simulink model "UAVSimulation"  (R2021b)
settings: Solver=VariableStepAuto  StartTime=0  StopTime=60  RelTol=1e-3
values from neighbouring files (symbols this model uses):
  m = 120000    [UAV_model.m]
  u1max = 25*pi/180    (= 0.436332312999)    [UAV_model.m]    (also in init.m; trim_values_straight_level.mat)
  u1min = -25*pi/180    (= -0.436332312999)    [UAV_model.m]    (also in init.m; trim_values_straight_level.mat)
  u2max = 10*pi/180    (= 0.174532925199)    [UAV_model.m]    (also in init.m; trim_values_straight_level.mat)
  u2min = -25*pi/180    (= -0.436332312999)    [UAV_model.m]    (also in init.m; trim_values_straight_level.mat)
  u4max = 10*pi/180    (= 0.174532925199)    [UAV_model.m]    (also in init.m; trim_values_straight_level.mat)
  u4min = 0.5*pi/180    (= 0.00872664625997)    [UAV_model.m]    (also in init.m; trim_values_straight_level.mat)
  u5max = 10*pi/180    (= 0.174532925199)    [UAV_model.m]    (also in init.m; trim_values_straight_level.mat)
  u5min = 0.5*pi/180    (= 0.00872664625997)    [UAV_model.m]    (also in init.m; trim_values_straight_level.mat)
  UStar = ZStar(10:14)    [UAV_trim.m]    (also in ValidateTrimPoint.m = temp.UStar; init.m = temp.UStar; trim_values_straight_level.mat = [0.000230087416011 -0.178007222496 0.000542025698534 0.08223)
  XStar = ZStar(1:9)    [UAV_trim.m]    (also in ValidateTrimPoint.m = temp.XStar; init.m = temp.XStar; trim_values_straight_level.mat = [84.9904926066 3.96412927226e-06 1.27128425211 2.6281652208e)
undefined symbols (not defined in the file or in its folder): Earth, ft, Payload, Receive, s, Send, UAV_model, WGS84
libraries: aerolibconvert2 x4, uavmavlinklib x4, simulink_extras x3, dspnetwork x3, aerolibfltsims x2, dspsigattribs x2, aerolibtransform2 x2, sensorgpslib x1, uavalgslib x1
settings Model: Creator=mikol  LastModifiedBy=mikol
settings SolverCC: AlgebraicLoopSolver=TrustRegion
settings DataIOCC: SaveFormat=StructureWithTime
settings OptimizationCC: BlockReduction=off  BufferReuse=off
settings DebuggingCC: AlgebraicLoopMsg=none  UnconnectedInputMsg=none  UnconnectedOutputMsg=none  UnconnectedLineMsg=none  SFMachineParentedDataDiag=warning
settings ExplorerConfigSet: SimMechanicsOpenEditorOnUpdate=off

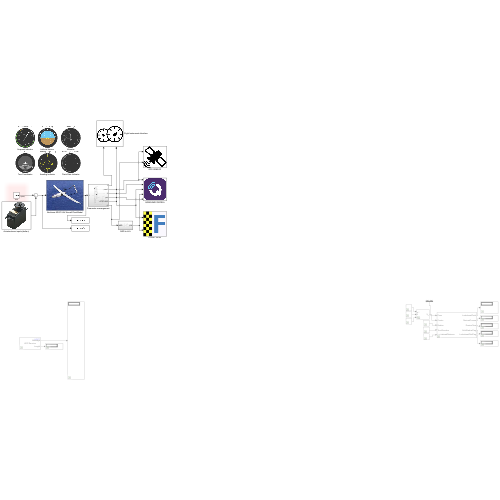
[thumbnail: Simulink's stored preview of the top-level diagram]
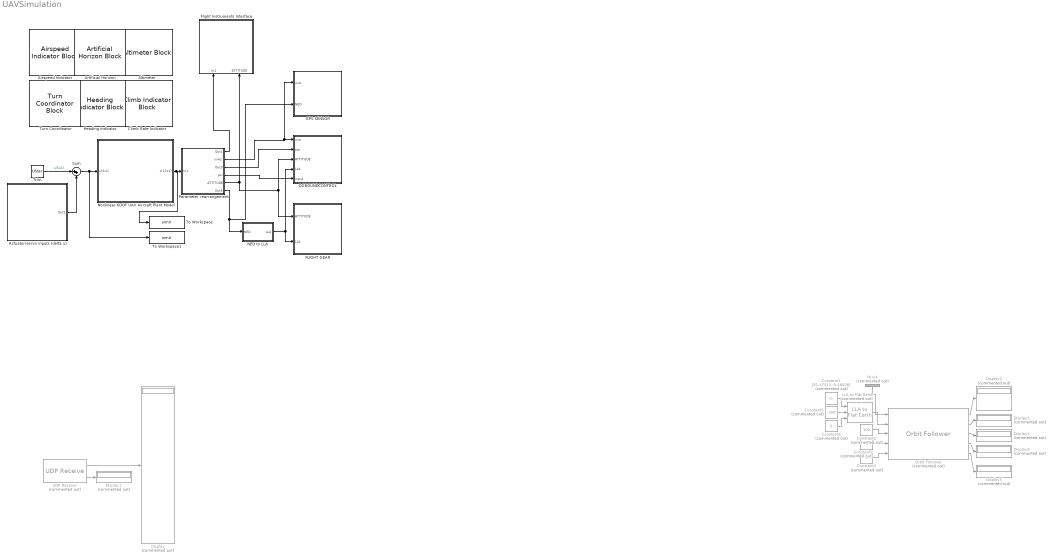
== system UAVSimulation ==
  Actuator/servo inputs (delta u) : Subsystem
      mask Display: image('FUTM0075_A0_R28XQZ28.jpg'); % Use "Edit Image" on toolstrip to change.
  Airspeed Indicator : AirspeedIndicatorBlock
  Altimeter : AltimeterBlock
  Artificial Horizon : ArtificialHorizonBlock
  Climb Rate Indicator : ClimbIndicatorBlock
  Constant1 : Constant  Commented=on  Value=[51.47413 -0.46008]
  Constant2 : Constant  Commented=on  Value=100
  Constant3 : Constant  Commented=on
  Constant4 : Constant  Commented=on  Value=5
  Constant5 : Constant  Commented=on  Value=-300
  Constant6 : Constant  Commented=on  Value=0
  Display{,1..6} (7 alike) : Display  Commented=on
  FLIGHT GEAR : Subsystem
      mask Display: image('icon.png'); % Use "Edit Image" on toolstrip to change.
  Flight Instruments Interface : Subsystem
      mask Display: image('167346-200.png'); % Use "Edit Image" on toolstrip to change.
  GPS SENSOR : Subsystem
      mask Display: image('gps.png'); % Use "Edit Image" on toolstrip to change.
  Heading Indicator : HeadingIndicatorBlock
  LLA to Flat Earth : aerolibtransform2/LLA to Flat Earth  Commented=on  units=Metric (MKS)  ptype=Earth (WGS84)  F=1/298.257223563  R=6378137  refPosPort=off  LL0=[51.47413 -0.46008]  psi=0
      settings: SourceProductBaseCode=AE
  Mux4 : Mux  Commented=on  Inputs=2
  NED to LLA : Subsystem
  Nonlinear 6DOF UAV Aircraft Plant Model : Subsystem
      mask Display: image('aerosonde-uav-bg.jpg'); % Use "Edit Image" on toolstrip to change.
  Orbit Follower : uavalgslib/Orbit Follower  Commented=on  UAVType=fixed-wing  MinOrbitRadius=1  MinLookaheadDistance=0.1  ExternalReset=none  ShowCrossTrackErrorOutput=off  ShowNumTurnsOutput=off  SimulateUsing=Interpreted execution
      settings: SourceProductBaseCode=UV
  Parameter rearrangement : Subsystem
  QGROUNDCONTROL : Subsystem
      mask Display: image('QGroundControl_App_Icon.png'); % Use "Edit Image" on toolstrip to change.
  Sum : Sum  Inputs=|++
  To Workspace : ToWorkspace  VariableName=simX  SaveFormat=Timeseries  SampleTime=-1
  To Workspace1 : ToWorkspace  VariableName=simU  SaveFormat=Timeseries  SampleTime=-1
  Trim : Constant  Value=UStar
  Turn Coordinator : TurnCoordinatorBlock
  UDP Receive : dspnetwork/UDP Receive  Commented=on  localURL='0.0.0.0'  localPort=14500  remoteURL='0.0.0.0'  remotePort=-1  recvBufferSize=8192  dims=263  signalDatatype=uint8  isComplex=off  isVarSize=off  showBlockingTime=on  blockingTime=0  sampletime=0.01  blockPlatform=HOST
  wires:
  Nonlinear 6DOF UAV Aircraft Plant Model/1(x(12x1)) -> To Workspace/1, Parameter rearrangement/1(In1)
  Trim/1 -> Sum/1  "u(5x1)"
  Actuator/servo inputs (delta u)/1(Out1) -> Sum/2
  Sum/1 -> To Workspace1/1, Nonlinear 6DOF UAV Aircraft Plant Model/1(u(5x1))
  UDP Receive/1 -> Display/1
  UDP Receive/2 -> Display1/1
  Mux4/1 -> Orbit Follower/1
  Constant4/1 -> Orbit Follower/5
  Orbit Follower/3 -> Display4/1
  Orbit Follower/1 -> Display2/1
  Orbit Follower/4 -> Display6/1
  Constant3/1 -> Orbit Follower/4
  Orbit Follower/2 -> Display3/1
  Constant5/1 -> LLA to Flat Earth/2
  Constant1/1 -> LLA to Flat Earth/1
  LLA to Flat Earth/1 -> Orbit Follower/2
  Constant2/1 -> Orbit Follower/3
  Orbit Follower/5 -> Display5/1
  Constant6/1 -> LLA to Flat Earth/3
  NED to LLA/1(LLA) -> FLIGHT GEAR/2(LLA), QGROUNDCONTROL/4(LLA)
  Parameter rearrangement/5(ATTITUDE) -> Flight Instruments Interface/2(ATTITUDE), FLIGHT GEAR/1(ATTITUDE), QGROUNDCONTROL/3(ATTITUDE)
  Parameter rearrangement/2(uvw1) -> GPS SENSOR/1(uvw), QGROUNDCONTROL/1(uvw)
  Parameter rearrangement/6(Out6) -> GPS SENSOR/2(NED), NED to LLA/1(NED)
  Parameter rearrangement/1(Out1) -> Flight Instruments Interface/1(In1)
  Parameter rearrangement/3(Out3) -> QGROUNDCONTROL/2(pqr)
  Parameter rearrangement/4(psi) -> QGROUNDCONTROL/5(Input)

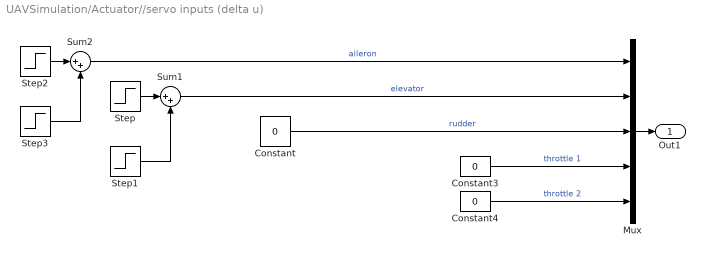
== system UAVSimulation/Actuator//servo inputs (delta u) ==
  Constant : Constant  Value=0
  Constant3 : Constant  Value=0
  Constant4 : Constant  Value=0
  Mux : Mux  Inputs=5
  Step : Step  Time=10  After=-5*pi/180  SampleTime=0
  Step1 : Step  Time=10+5  After=5*pi/180  SampleTime=0
  Step2 : Step  Time=15  After=-5*pi/180  SampleTime=0
  Step3 : Step  Time=15+20  After=5*pi/180  SampleTime=0
  Sum1 : Sum  Inputs=|++
  Sum2 : Sum  Inputs=|++
  Out1 : Outport
  wires:
  Step/1 -> Sum1/1
  Constant/1 -> Mux/3  "rudder"
  Constant4/1 -> Mux/5  "throttle 2"
  Step1/1 -> Sum1/2
  Constant3/1 -> Mux/4  "throttle 1"
  Mux/1 -> Out1/1
  Sum2/1 -> Mux/1  "aileron"
  Sum1/1 -> Mux/2  "elevator"
  Step2/1 -> Sum2/1
  Step3/1 -> Sum2/2

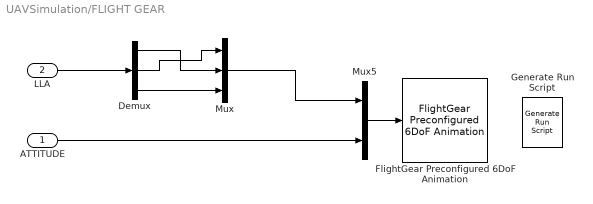
== system UAVSimulation/FLIGHT GEAR ==
  ATTITUDE : Inport
  LLA : Inport  Port=2
  Demux : Demux  Outputs=3
  FlightGear Preconfigured 6DoF Animation : aerolibfltsims/FlightGear Preconfigured 6DoF Animation  xFlightGearVersion=v2019.1  DestinationIpAddress=127.0.0.1  DestinationPort=5502  SampleTime=1/30  packetVersion=24
  Generate Run Script : aerolibfltsims/Generate Run Script  Architecture=Win64  dataFlow=Send-Receive  GeometryModelName=c172p  AirportId=KSFO  RunwayId=10L  InitialAltitude=7224  InitialHeading=113  OffsetDistance=4.72  OffsetAzimuth=0  InstallScenery=on  DisableShaders=on  OriginAddress=127.0.0.1  DestinationPort=5502  OriginPort=5505  LocalAddress=127.0.0.1  OutputFileName=runfg.bat  FlightGearBaseDirectory=D:\Program Files\FlightGear 2020.3
  Mux : Mux  Inputs=3
  Mux5 : Mux  Inputs=2
  wires:
  Mux5/1 -> FlightGear Preconfigured 6DoF Animation/1
  ATTITUDE/1 -> Mux5/2
  Mux/1 -> Mux5/1
  LLA/1 -> Demux/1
  Demux/1 -> Mux/2
  Demux/2 -> Mux/1
  Demux/3 -> Mux/3

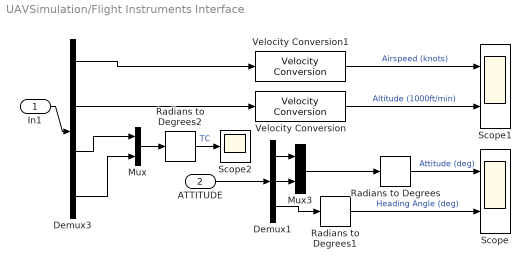
== system UAVSimulation/Flight Instruments Interface ==
  In1 : Inport
  ATTITUDE : Inport  Port=2
  Demux1 : Demux  Outputs=3
  Demux3 : Demux
  Mux : Mux  Inputs=2
  Mux3 : Mux  Inputs=2
  Radians to Degrees : simulink_extras/Transformations/Radians to Degrees
  Radians to Degrees1 : simulink_extras/Transformations/Radians to Degrees
  Radians to Degrees2 : simulink_extras/Transformations/Radians to Degrees
  Scope : Scope  NumInputPorts=2
  Scope1 : Scope  NumInputPorts=2
  Scope2 : Scope
  Velocity Conversion : aerolibconvert2/Velocity Conversion  IU=m/s  OU=ft/min
  Velocity Conversion1 : aerolibconvert2/Velocity Conversion  IU=m/s  OU=kts
  wires:
  Velocity Conversion1/1 -> Scope1/1  "Airspeed (knots)"
  Demux1/2 -> Mux3/2
  In1/1 -> Demux3/1
  Demux1/3 -> Radians to Degrees1/1
  Demux3/2 -> Velocity Conversion/1
  Mux3/1 -> Radians to Degrees/1
  Radians to Degrees/1 -> Scope/1  "Attitude (deg)"
  Radians to Degrees1/1 -> Scope/2  "Heading Angle (deg)"
  Velocity Conversion/1 -> Scope1/2  "Altitude (1000ft/min)"
  Demux1/1 -> Mux3/1
  Radians to Degrees2/1 -> Scope2/1  "TC"
  Mux/1 -> Radians to Degrees2/1
  Demux3/3 -> Mux/1
  Demux3/4 -> Mux/2
  Demux3/1 -> Velocity Conversion1/1
  ATTITUDE/1 -> Demux1/1

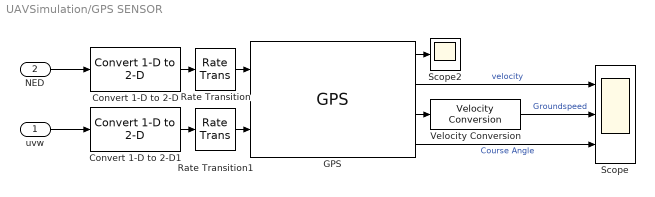
== system UAVSimulation/GPS SENSOR ==
  uvw : Inport
  NED : Inport  Port=2
  Convert 1-D to 2-D : dspsigattribs/Convert 1-D to 2-D  M=1  N=3  frameBasedOut=off
      settings: SourceProductBaseCode=DS
  Convert 1-D to 2-D1 : dspsigattribs/Convert 1-D to 2-D  M=1  N=3  frameBasedOut=off
      settings: SourceProductBaseCode=DS
  GPS : sensorgpslib/GPS  DispRefFrame=NED  PositionInputFormat=Geodetic  ReferenceLocation=[ 0, 0, 0 ]  HorizontalPositionAccuracy=1.6  VerticalPositionAccuracy=3  VelocityAccuracy=0.1  DecayFactor=0.999  SeedDouble=67  SimulateUsing=Interpreted execution
      settings: SourceProductBaseCode=TF,NV,UV
  Rate Transition : RateTransition  OutPortSampleTime=0.2
  Rate Transition1 : RateTransition  OutPortSampleTime=0.2
  Scope : Scope  NumInputPorts=3
  Scope2 : Scope
  Velocity Conversion : aerolibconvert2/Velocity Conversion  IU=m/s  OU=kts
  wires:
  GPS/3 -> Velocity Conversion/1
  Convert 1-D to 2-D/1 -> Rate Transition/1
  Rate Transition1/1 -> GPS/2
  GPS/1 -> Scope2/1
  Rate Transition/1 -> GPS/1
  GPS/4 -> Scope/3  "Course Angle"
  Convert 1-D to 2-D1/1 -> Rate Transition1/1
  GPS/2 -> Scope/1  "velocity"
  Velocity Conversion/1 -> Scope/2  "Groundspeed"
  uvw/1 -> Convert 1-D to 2-D1/1
  NED/1 -> Convert 1-D to 2-D/1

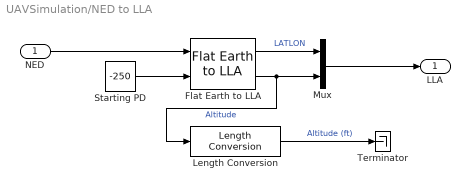
== system UAVSimulation/NED to LLA ==
  NED : Inport
  Flat Earth to LLA : aerolibtransform2/Flat Earth to LLA  units=Metric (MKS)  ptype=Earth (WGS84)  F=1/298.257223563  R=6378137  refPosPort=off  LL0=[51.47413 -0.46008]  psi=0
  Length Conversion : aerolibconvert2/Length Conversion  IU=m  OU=ft
  Mux : Mux  Inputs=2
  Starting PD : Constant  Value=-250
  Terminator : Terminator
  LLA : Outport
  wires:
  Starting PD/1 -> Flat Earth to LLA/2
  NED/1 -> Flat Earth to LLA/1
  Flat Earth to LLA/1 -> Mux/1  "LATLON"
  Flat Earth to LLA/2 -> Length Conversion/1, Mux/2  "Altitude"
  Mux/1 -> LLA/1
  Length Conversion/1 -> Terminator/1  "Altitude (ft)"

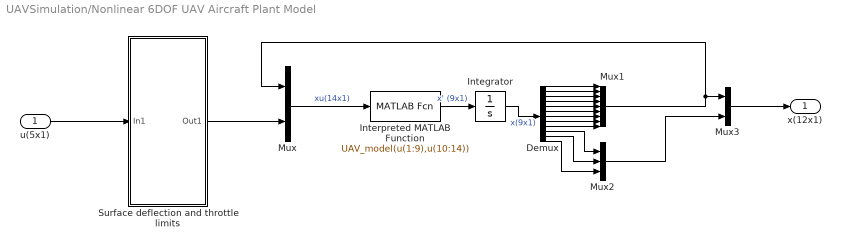
== system UAVSimulation/Nonlinear 6DOF UAV Aircraft Plant Model ==
  u(5x1) : Inport
  Demux : Demux  Outputs=12
  Integrator : Integrator  InitialCondition=XStar
  Interpreted MATLAB Function : MATLABFcn  MATLABFcn=UAV_model(u(1:9),u(10:14))
  Mux : Mux  Inputs=2
  Mux1 : Mux  Inputs=9
  Mux2 : Mux  Inputs=3
  Mux3 : Mux  Inputs=2
  Surface deflection and throttle limits : Subsystem
  x(12x1) : Outport
  wires:
  Mux/1 -> Interpreted MATLAB Function/1  "xu(14x1)"
  Interpreted MATLAB Function/1 -> Integrator/1  "x' (9x1)"
  u(5x1)/1 -> Surface deflection and throttle limits/1(In1)
  Surface deflection and throttle limits/1(Out1) -> Mux/2
  Demux/1 -> Mux1/1
  Demux/2 -> Mux1/2
  Demux/3 -> Mux1/3
  Demux/4 -> Mux1/4
  Demux/5 -> Mux1/5
  Demux/6 -> Mux1/6
  Demux/7 -> Mux1/7
  Demux/8 -> Mux1/8
  Demux/9 -> Mux1/9
  Demux/10 -> Mux2/1
  Demux/11 -> Mux2/2
  Demux/12 -> Mux2/3
  Mux2/1 -> Mux3/2
  Mux3/1 -> x(12x1)/1
  Integrator/1 -> Demux/1  "x(9x1)"
  Mux1/1 -> Mux/1, Mux3/1

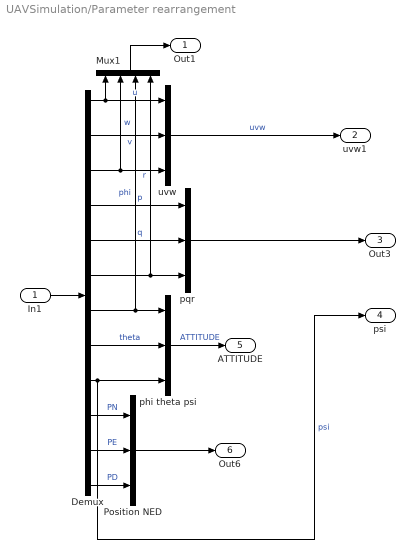
== system UAVSimulation/Parameter rearrangement ==
  In1 : Inport
  Demux : Demux  Outputs=12
  Mux1 : Mux
  Position NED : Mux  Inputs=3
  phi theta psi : Mux  Inputs=3
  pqr : Mux  Inputs=3
  uvw : Mux  Inputs=3
  Out1 : Outport
  uvw1 : Outport  Port=2
  Out3 : Outport  Port=3
  psi : Outport  Port=4
  ATTITUDE : Outport  Port=5
  Out6 : Outport  Port=6
  wires:
  Demux/9 -> phi theta psi/3, psi/1  "psi"
  Demux/5 -> pqr/2  "q"
  Demux/3 -> Mux1/2, uvw/3  "w"
  Demux/10 -> Position NED/1  "PN"
  Demux/1 -> uvw/1, Mux1/1  "u"
  Demux/7 -> phi theta psi/1, Mux1/3  "phi"
  Demux/11 -> Position NED/2  "PE"
  Demux/8 -> phi theta psi/2  "theta"
  Demux/2 -> uvw/2  "v"
  uvw/1 -> uvw1/1  "uvw"
  Demux/12 -> Position NED/3  "PD"
  Demux/4 -> pqr/1  "p"
  Demux/6 -> pqr/3, Mux1/4  "r"
  phi theta psi/1 -> ATTITUDE/1  "ATTITUDE"
  In1/1 -> Demux/1
  pqr/1 -> Out3/1
  Position NED/1 -> Out6/1
  Mux1/1 -> Out1/1

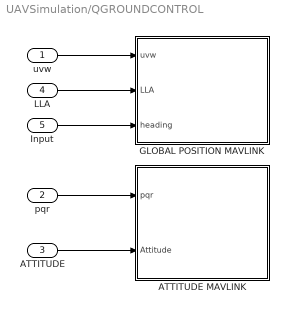
== system UAVSimulation/QGROUNDCONTROL ==
  uvw : Inport
  pqr : Inport  Port=2
  ATTITUDE : Inport  Port=3
  LLA : Inport  Port=4
  Input : Inport  Port=5
  ATTITUDE MAVLINK : Subsystem
  GLOBAL POSITION MAVLINK : Subsystem
  wires:
  uvw/1 -> GLOBAL POSITION MAVLINK/1(uvw)
  pqr/1 -> ATTITUDE MAVLINK/1(pqr)
  ATTITUDE/1 -> ATTITUDE MAVLINK/2(Attitude)
  LLA/1 -> GLOBAL POSITION MAVLINK/2(LLA)
  Input/1 -> GLOBAL POSITION MAVLINK/3(heading)

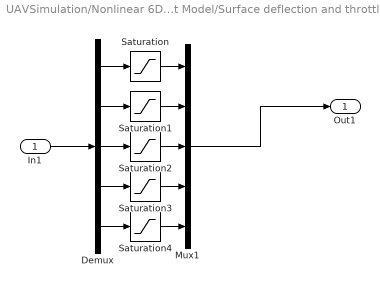
== system UAVSimulation/Nonlinear 6DOF UAV Aircraft Plant Model/Surface deflection and throttle limits ==
  In1 : Inport
  Demux : Demux  Outputs=5
  Mux1 : Mux  Inputs=5
  Saturation : Saturate  UpperLimit=u1max  LowerLimit=u1min
  Saturation1 : Saturate  UpperLimit=u2max  LowerLimit=u2min
  Saturation2 : Saturate  UpperLimit=u1max  LowerLimit=u1min
  Saturation3 : Saturate  UpperLimit=u4max  LowerLimit=u4min
  Saturation4 : Saturate  UpperLimit=u5max  LowerLimit=u5min
  Out1 : Outport
  wires:
  Demux/2 -> Saturation1/1
  Demux/3 -> Saturation2/1
  Saturation3/1 -> Mux1/4
  Saturation4/1 -> Mux1/5
  Saturation/1 -> Mux1/1
  Demux/1 -> Saturation/1
  Demux/4 -> Saturation3/1
  In1/1 -> Demux/1
  Saturation2/1 -> Mux1/3
  Demux/5 -> Saturation4/1
  Saturation1/1 -> Mux1/2
  Mux1/1 -> Out1/1

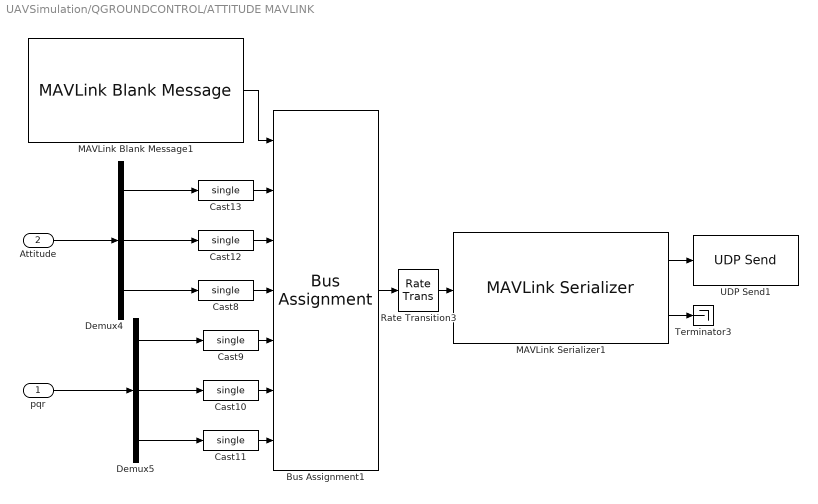
== system UAVSimulation/QGROUNDCONTROL/ATTITUDE MAVLINK ==
  pqr : Inport
  Attitude : Inport  Port=2
  Bus Assignment1 : BusAssignment  AssignedSignals=Payload.roll,Payload.pitch,Payload.yaw,Payload.rollspeed,Payload.pitchspeed,Payload.yawspeed
  Cast{8..13} (6 alike) : DataTypeConversion  OutDataTypeStr=single
  Demux4 : Demux  Outputs=3
  Demux5 : Demux  Outputs=3
  MAVLink Blank Message1 : uavmavlinklib/MAVLink Blank Message  dialectSource=Select from standard MAVLink dialects  dialect=common.xml  dialectCustom=common.xml  version=2  messageType=ATTITUDE  SystemID=1  ComponentID=1  SampleTime=inf
      settings: SourceProductBaseCode=UV
  MAVLink Serializer1 : uavmavlinklib/MAVLink Serializer  dialectSource=Select from standard MAVLink dialects  dialect=common.xml  dialectCustom=common.xml  version=2  messageType=ATTITUDE
      settings: SourceProductBaseCode=UV
  Rate Transition3 : RateTransition  OutPortSampleTime=0.1
  Terminator3 : Terminator
  UDP Send1 : dspnetwork/UDP Send  remoteURL='127.0.0.1'  remotePort=qgcPort  localURL='0.0.0.0'  localPortSource=Automatically determine  localPort=-1  sendBufferSize=8192  sampletime=-1  blockPlatform=[]  separateLengthPort=0
  wires:
  Demux4/2 -> Cast12/1
  Cast11/1 -> Bus Assignment1/7
  Cast8/1 -> Bus Assignment1/4
  MAVLink Blank Message1/1 -> Bus Assignment1/1
  MAVLink Serializer1/1 -> UDP Send1/1
  Demux4/1 -> Cast13/1
  Demux5/2 -> Cast10/1
  Cast12/1 -> Bus Assignment1/3
  MAVLink Serializer1/2 -> Terminator3/1
  Cast13/1 -> Bus Assignment1/2
  Cast9/1 -> Bus Assignment1/5
  Bus Assignment1/1 -> Rate Transition3/1
  Demux4/3 -> Cast8/1
  Demux5/1 -> Cast9/1
  Cast10/1 -> Bus Assignment1/6
  Demux5/3 -> Cast11/1
  Rate Transition3/1 -> MAVLink Serializer1/1
  Attitude/1 -> Demux4/1
  pqr/1 -> Demux5/1

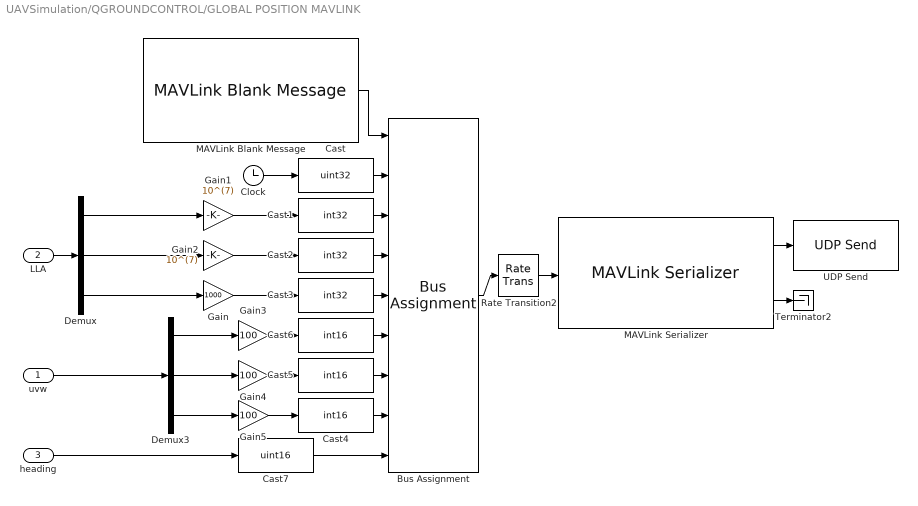
== system UAVSimulation/QGROUNDCONTROL/GLOBAL POSITION MAVLINK ==
  uvw : Inport
  LLA : Inport  Port=2
  heading : Inport  Port=3
  Bus Assignment : BusAssignment  AssignedSignals=Payload.time_boot_ms,Payload.lat,Payload.lon,Payload.relative_alt,Payload.vx,Payload.vy,Payload.vz,Payload.hdg
  Cast : DataTypeConversion  OutDataTypeStr=uint32
  Cast1 : DataTypeConversion  OutDataTypeStr=int32
  Cast2 : DataTypeConversion  OutDataTypeStr=int32
  Cast3 : DataTypeConversion  OutDataTypeStr=int32
  Cast4 : DataTypeConversion  OutDataTypeStr=int16
  Cast5 : DataTypeConversion  OutDataTypeStr=int16
  Cast6 : DataTypeConversion  OutDataTypeStr=int16
  Cast7 : DataTypeConversion  OutDataTypeStr=uint16
  Clock : Clock
  Demux : Demux  Outputs=3
  Demux3 : Demux  Outputs=3
  Gain : Gain  Gain=1000
  Gain1 : Gain  Gain=10^(7)
  Gain2 : Gain  Gain=10^(7)
  Gain3 : Gain  Gain=100
  Gain4 : Gain  Gain=100
  Gain5 : Gain  Gain=100
  MAVLink Blank Message : uavmavlinklib/MAVLink Blank Message  dialectSource=Select from standard MAVLink dialects  dialect=common.xml  dialectCustom=common.xml  version=2  messageType=GLOBAL_POSITION_INT  SystemID=1  ComponentID=1  SampleTime=inf
      settings: SourceProductBaseCode=UV
  MAVLink Serializer : uavmavlinklib/MAVLink Serializer  dialectSource=Select from standard MAVLink dialects  dialect=common.xml  dialectCustom=common.xml  version=2  messageType=GLOBAL_POSITION_INT
      settings: SourceProductBaseCode=UV
  Rate Transition2 : RateTransition  OutPortSampleTime=0.1
  Terminator2 : Terminator
  UDP Send : dspnetwork/UDP Send  remoteURL='127.0.0.1'  remotePort=qgcPort  localURL='0.0.0.0'  localPortSource=Automatically determine  localPort=-1  sendBufferSize=8192  sampletime=-1  blockPlatform=[]  separateLengthPort=0
  wires:
  MAVLink Blank Message/1 -> Bus Assignment/1
  Cast6/1 -> Bus Assignment/6
  Cast3/1 -> Bus Assignment/5
  Cast1/1 -> Bus Assignment/3
  Cast4/1 -> Bus Assignment/8
  MAVLink Serializer/2 -> Terminator2/1
  Cast5/1 -> Bus Assignment/7
  Clock/1 -> Cast/1
  Demux3/3 -> Gain5/1
  Cast2/1 -> Bus Assignment/4
  MAVLink Serializer/1 -> UDP Send/1
  Demux3/2 -> Gain4/1
  Bus Assignment/1 -> Rate Transition2/1
  Gain2/1 -> Cast2/1
  Gain1/1 -> Cast1/1
  Cast/1 -> Bus Assignment/2
  Rate Transition2/1 -> MAVLink Serializer/1
  uvw/1 -> Demux3/1
  Demux/2 -> Gain2/1
  Demux/1 -> Gain1/1
  LLA/1 -> Demux/1
  Gain/1 -> Cast3/1
  Demux/3 -> Gain/1
  Cast7/1 -> Bus Assignment/9
  heading/1 -> Cast7/1
  Gain5/1 -> Cast4/1
  Gain4/1 -> Cast5/1
  Demux3/1 -> Gain3/1
  Gain3/1 -> Cast6/1
